simulink model "sampleModel1000"  (R2022a)
settings: Solver=VariableStepAuto  StartTime=0.0  StopTime=10.0  RelTol=1e-3
undefined symbols (not defined in the file): DiscIntNeverNeededParam, magnitude, Newton, Raphson
libraries: simulink x216, slpidlib x76
(part 3 of 10)

== system sampleModel1000/cfblk162 ==
  cfblk1 : Inport
  cfblk14 : Inport  Port=2
  cfblk10 : Subsystem
  cfblk11 : Subsystem
  cfblk12 : Subsystem
  cfblk13 : Subsystem
  cfblk{16..19} (4 alike) : Delay  SampleTime=1
  cfblk3 : slpidlib/PID Controller (2DOF)  Controller=PID  Form=Parallel  TimeDomain=Discrete-time  UseExternalTs=off  SampleTime=1  IntegratorMethod=Forward Euler  FilterMethod=Forward Euler  ControllerParametersSource=internal  P=1  I=1  UseKiTs=off  D=0  N=100  UseFilter=on  b=1  c=1  TunerSelectOption=Transfer Function Based (PID Tuner App)  InitialConditionSource=internal  InitialConditionForIntegrator=0  InitialConditionForFilter=0  DifferentiatorICPrevScaledInput=0  ExternalReset=none  TrackingMode=off  Kt=1  LimitOutput=off  SatLimitsSource=internal  UpperSaturationLimit=inf  LowerSaturationLimit=-inf  LinearizeAsGain=off  AntiWindupMode=none  Kb=1  POutMin=[]  POutMax=[]  IOutMin=[]  IOutMax=[]  DOutMin=[]  DOutMax=[]  NOutMin=[]  NOutMax=[]  bOutMin=[]  bOutMax=[]  cOutMin=[]  cOutMax=[]  SumOutMin=[]  SumOutMax=[]  SaturationOutMin=[]  SaturationOutMax=[]  PParamMin=[]  PParamMax=[]  IParamMin=[]  IParamMax=[]  DParamMin=[]  DParamMax=[]  NParamMin=[]  NParamMax=[]  bParamMin=[]  bParamMax=[]  cParamMin=[]  cParamMax=[]  KbParamMin=[]  KbParamMax=[]  KtParamMin=[]  KtParamMax=[]  KbOutMin=[]  KbOutMax=[]  KtOutMin=[]  KtOutMax=[]  IntegratorOutMin=[]  IntegratorOutMax=[]  FilterOutMin=[]  FilterOutMax=[]  SumI1OutMin=[]  SumI1OutMax=[]  SumI2OutMin=[]  SumI2OutMax=[]  SumI3OutMin=[]  SumI3OutMax=[]  SumI4OutMin=[]  SumI4OutMax=[]  SumDOutMin=[]  SumDOutMax=[]  Sum1OutMin=[]  Sum1OutMax=[]  Sum2OutMin=[]  Sum2OutMax=[]  Sum3OutMin=[]  Sum3OutMax=[]  DifferentiatorOutMin=[]  DifferentiatorOutMax=[]  FilterDiffOutCoefMin=[]  FilterDiffOutCoefMax=[]  ReciprocalOutMin=[]  ReciprocalOutMax=[]  SumDenOutMin=[]  SumDenOutMax=[]  SumNumOutMin=[]  SumNumOutMax=[]  DivideOutMin=[]  DivideOutMax=[]  UdiffTsProdOutMin=[]  UdiffTsProdOutMax=[]  NTsProdOutMin=[]  NTsProdOutMax=[]  UintegralTsProdOutMin=[]  UintegralTsProdOutMax=[]  UngainTsProdOutMin=[]  UngainTsProdOutMax=[]  IntegratorContinuousStateAttributes=''  IntegratorStateMustResolveToSignalObject=off  IntegratorRTWStateStorageClass=Auto  FilterContinuousStateAttributes=''  FilterStateMustResolveToSignalObject=off  FilterRTWStateStorageClass=Auto  ParallelPVariant=InternalParameters  IdealPVariant=Disabled  IVariant=InternalParameters  DVariant=InternalParameters  bVariant=InternalParameters  cVariant=InternalParameters  IntegratorVariant=Discrete  SatVariant=Disabled  AWVariant=Passthrough  PCopyVariant=Disabled  TRVariant=Disabled  FdbkBlocksVariant=Forward  IdealPFdbkVariant=Disabled  SatFdbkVariant=Disabled  DerivativeFilterVariant=ForwardEulerFilter  NVariant=InternalParameters  NCopyVariant=Disabled  FilterICVariant=InternalICsFilter  IntegratorICVariant=InternalICs  ExternalResetVariant=Disabled  TRSumVariant=Passthrough  SumFdbkVariant=Disabled  SumVariant=Sum_PID  TsampFilterVariant=InternalTs  TsampNgainVariant=Passthrough  TsampIntegralVariant=Passthrough  ExternalSaturationOutDataTypeStr=Inherit: Same as second input
      settings: SourceProductBaseCode=SL
  cfblk4 : simulink/Discrete/Transfer Fcn First Order  PoleZ=0.95  ICPrevOutput=0.0  DoSatur=off
  cfblk5 : ComplexToMagnitudeAngle
  cfblk6 : Sum  Inputs=+-
  cfblk7 : Abs  SaturateOnIntegerOverflow=off
  cfblk8 : Rounding
  cfblk9 : Constant  Value=[225906652.287028]  SampleTime=1
  cfblk2 : Outport
  cfblk15 : Outport  Port=2
  wires:
  cfblk13/1(cfblk2) -> cfblk3/1, cfblk11/4(cfblk13)
  cfblk10/1(cfblk2) -> cfblk8/1
  cfblk6/1 -> cfblk15/1
  cfblk3/1 -> cfblk4/1
  cfblk7/1 -> cfblk5/1, cfblk18/1
  cfblk9/1 -> cfblk3/2
  cfblk1/1 -> cfblk6/1, cfblk12/3(cfblk8)
  cfblk12/1(cfblk2) -> cfblk13/2(cfblk7)
  cfblk10/2(cfblk15) -> cfblk11/1(cfblk1)
  cfblk8/1 -> cfblk2/1
  cfblk5/2 -> cfblk11/2(cfblk11), cfblk11/3(cfblk12)
  cfblk4/1 -> cfblk10/2(cfblk13)
  cfblk14/1 -> cfblk13/3(cfblk8), cfblk12/4(cfblk9)
  cfblk10/3(cfblk16) -> cfblk7/1
  cfblk12/2(cfblk10) -> cfblk10/3(cfblk14)
  cfblk12/3(cfblk11) -> cfblk6/2
  cfblk11/1(cfblk2) -> cfblk16/1
  cfblk16/1 -> cfblk12/2(cfblk7)
  cfblk11/2(cfblk14) -> cfblk17/1
  cfblk17/1 -> cfblk10/1(cfblk1)
  cfblk18/1 -> cfblk12/1(cfblk1)
  cfblk5/1 -> cfblk19/1
  cfblk19/1 -> cfblk13/1(cfblk1)

== system sampleModel1000/cfblk163 ==
  cfblk1 : Inport
  cfblk10 : Delay  SampleTime=1
  cfblk11 : Delay  SampleTime=1
  cfblk3 : slpidlib/PID Controller (2DOF)  Controller=PID  Form=Parallel  TimeDomain=Discrete-time  UseExternalTs=off  SampleTime=1  IntegratorMethod=Forward Euler  FilterMethod=Forward Euler  ControllerParametersSource=internal  P=1  I=1  UseKiTs=off  D=0  N=100  UseFilter=on  b=1  c=1  TunerSelectOption=Transfer Function Based (PID Tuner App)  InitialConditionSource=internal  InitialConditionForIntegrator=0  InitialConditionForFilter=0  DifferentiatorICPrevScaledInput=0  ExternalReset=none  TrackingMode=off  Kt=1  LimitOutput=off  SatLimitsSource=internal  UpperSaturationLimit=inf  LowerSaturationLimit=-inf  LinearizeAsGain=off  AntiWindupMode=none  Kb=1  POutMin=[]  POutMax=[]  IOutMin=[]  IOutMax=[]  DOutMin=[]  DOutMax=[]  NOutMin=[]  NOutMax=[]  bOutMin=[]  bOutMax=[]  cOutMin=[]  cOutMax=[]  SumOutMin=[]  SumOutMax=[]  SaturationOutMin=[]  SaturationOutMax=[]  PParamMin=[]  PParamMax=[]  IParamMin=[]  IParamMax=[]  DParamMin=[]  DParamMax=[]  NParamMin=[]  NParamMax=[]  bParamMin=[]  bParamMax=[]  cParamMin=[]  cParamMax=[]  KbParamMin=[]  KbParamMax=[]  KtParamMin=[]  KtParamMax=[]  KbOutMin=[]  KbOutMax=[]  KtOutMin=[]  KtOutMax=[]  IntegratorOutMin=[]  IntegratorOutMax=[]  FilterOutMin=[]  FilterOutMax=[]  SumI1OutMin=[]  SumI1OutMax=[]  SumI2OutMin=[]  SumI2OutMax=[]  SumI3OutMin=[]  SumI3OutMax=[]  SumI4OutMin=[]  SumI4OutMax=[]  SumDOutMin=[]  SumDOutMax=[]  Sum1OutMin=[]  Sum1OutMax=[]  Sum2OutMin=[]  Sum2OutMax=[]  Sum3OutMin=[]  Sum3OutMax=[]  DifferentiatorOutMin=[]  DifferentiatorOutMax=[]  FilterDiffOutCoefMin=[]  FilterDiffOutCoefMax=[]  ReciprocalOutMin=[]  ReciprocalOutMax=[]  SumDenOutMin=[]  SumDenOutMax=[]  SumNumOutMin=[]  SumNumOutMax=[]  DivideOutMin=[]  DivideOutMax=[]  UdiffTsProdOutMin=[]  UdiffTsProdOutMax=[]  NTsProdOutMin=[]  NTsProdOutMax=[]  UintegralTsProdOutMin=[]  UintegralTsProdOutMax=[]  UngainTsProdOutMin=[]  UngainTsProdOutMax=[]  IntegratorContinuousStateAttributes=''  IntegratorStateMustResolveToSignalObject=off  IntegratorRTWStateStorageClass=Auto  FilterContinuousStateAttributes=''  FilterStateMustResolveToSignalObject=off  FilterRTWStateStorageClass=Auto  ParallelPVariant=InternalParameters  IdealPVariant=Disabled  IVariant=InternalParameters  DVariant=InternalParameters  bVariant=InternalParameters  cVariant=InternalParameters  IntegratorVariant=Discrete  SatVariant=Disabled  AWVariant=Passthrough  PCopyVariant=Disabled  TRVariant=Disabled  FdbkBlocksVariant=Forward  IdealPFdbkVariant=Disabled  SatFdbkVariant=Disabled  DerivativeFilterVariant=ForwardEulerFilter  NVariant=InternalParameters  NCopyVariant=Disabled  FilterICVariant=InternalICsFilter  IntegratorICVariant=InternalICs  ExternalResetVariant=Disabled  TRSumVariant=Passthrough  SumFdbkVariant=Disabled  SumVariant=Sum_PID  TsampFilterVariant=InternalTs  TsampNgainVariant=Passthrough  TsampIntegralVariant=Passthrough  ExternalSaturationOutDataTypeStr=Inherit: Same as second input
      settings: SourceProductBaseCode=SL
  cfblk4 : DiscreteFir  SampleTime=1
  cfblk5 : ComplexToRealImag
  cfblk6 : DotProduct  OutDataTypeStr=Inherit: Inherit via internal rule
  cfblk7 : Subsystem
  cfblk8 : Subsystem
  cfblk9 : Delay  SampleTime=1
  cfblk2 : Outport
  wires:
  cfblk3/1 -> cfblk8/1(cfblk1)
  cfblk6/1 -> cfblk7/1(cfblk1), cfblk3/2
  cfblk1/1 -> cfblk6/1
  cfblk4/1 -> cfblk2/1
  cfblk7/1(cfblk2) -> cfblk8/2(cfblk6)
  cfblk8/1(cfblk2) -> cfblk5/1
  cfblk7/2(cfblk8) -> cfblk4/1
  cfblk7/3(cfblk9) -> cfblk3/1
  cfblk5/1 -> cfblk9/1
  cfblk9/1 -> cfblk6/2
  cfblk5/2 -> cfblk10/1
  cfblk10/1 -> cfblk8/3(cfblk7)
  cfblk8/2(cfblk8) -> cfblk11/1
  cfblk11/1 -> cfblk7/2(cfblk7)

== system sampleModel1000/cfblk164 ==
  cfblk1 : Inport
  cfblk8 : Inport  Port=2
  cfblk10 : Subsystem  TreatAsAtomicUnit=on
  cfblk11 : Subsystem  TreatAsAtomicUnit=on
  cfblk12 : Delay  SampleTime=1
  cfblk3 : simulink/Math Operations/MinMax Running Resettable  Function=min  vinit=0.0
  cfblk4 : Sqrt  Operator=rSqrt  AlgorithmType=Newton-Raphson
  cfblk5 : Constant  Value=[165198451.789019]  SampleTime=1
  cfblk6 : Subsystem
  cfblk7 : If  IfExpression=u1 >= 0  SampleTime=1
  cfblk2 : Outport
  cfblk9 : Outport  Port=2
  wires:
  cfblk3/1 -> cfblk2/1
  cfblk8/1 -> cfblk4/1
  cfblk5/1 -> cfblk9/1, cfblk10/2(cfblk9)
  cfblk6/1(cfblk2) -> cfblk11/1(cfblk1)
  cfblk6/2(cfblk10) -> cfblk7/1
  cfblk6/3(cfblk11) -> cfblk3/1
  cfblk1/1 -> cfblk3/2
  cfblk4/1 -> cfblk6/2(cfblk9), cfblk10/3(cfblk10)
  cfblk11/1(cfblk2) -> cfblk10/1(cfblk1)
  cfblk7/1 -> cfblk10/Action
  cfblk7/2 -> cfblk11/Action
  cfblk10/1(cfblk2) -> cfblk12/1
  cfblk12/1 -> cfblk6/1(cfblk1)

== system sampleModel1000/cfblk165 ==
  cfblk1 : Inport
  cfblk10 : Subsystem
  cfblk11 : Subsystem
  cfblk12 : Subsystem
  cfblk13 : Subsystem
  cfblk15 : Delay  SampleTime=1
  cfblk3 : DiscreteStateSpace
  cfblk4 : Delay  SampleTime=1
  cfblk5 : Sum  Inputs=+
  cfblk6 : Constant  Value=[-942559068.084859]  SampleTime=1
  cfblk7 : Constant  Value=[883886855.435224]  SampleTime=1
  cfblk8 : Constant  Value=[497965959.676924]  SampleTime=1
  cfblk9 : Constant  Value=[-864930801.055590]  SampleTime=1
  cfblk2 : Outport
  cfblk14 : Outport  Port=2
  wires:
  cfblk7/1 -> cfblk5/1
  cfblk4/1 -> cfblk12/1(cfblk1)
  cfblk1/1 -> cfblk10/1(cfblk1)
  cfblk5/1 -> cfblk10/2(cfblk6)
  cfblk3/1 -> cfblk13/1(cfblk1), cfblk13/2(cfblk9)
  cfblk9/1 -> cfblk10/3(cfblk7)
  cfblk11/1(cfblk2) -> cfblk3/1
  cfblk6/1 -> cfblk11/1(cfblk1), cfblk2/1
  cfblk12/1(cfblk2) -> cfblk14/1
  cfblk8/1 -> cfblk11/2(cfblk16)
  cfblk12/2(cfblk16) -> cfblk11/3(cfblk17)
  cfblk10/1(cfblk2) -> cfblk4/1
  cfblk13/1(cfblk2) -> cfblk15/1
  cfblk15/1 -> cfblk12/2(cfblk15)

== system sampleModel1000/cfblk166 ==
  cfblk1 : Inport
  cfblk10 : Subsystem
  cfblk11 : Subsystem
  cfblk{12..16} (5 alike) : Delay  SampleTime=1
  cfblk3 : simulink/Discrete/Transfer Fcn Real Zero  ZeroZ=0.75  ICPrevInput=0.0  DoSatur=off
      settings: SourceProductBaseCode=SL
  cfblk4 : simulink/Discrete/Transfer Fcn First Order  PoleZ=0.95  ICPrevOutput=0.0  DoSatur=off
  cfblk5 : slpidlib/PID Controller (2DOF)  Controller=PID  Form=Parallel  TimeDomain=Discrete-time  UseExternalTs=off  SampleTime=1  IntegratorMethod=Forward Euler  FilterMethod=Forward Euler  ControllerParametersSource=internal  P=1  I=1  UseKiTs=off  D=0  N=100  UseFilter=on  b=1  c=1  TunerSelectOption=Transfer Function Based (PID Tuner App)  InitialConditionSource=internal  InitialConditionForIntegrator=0  InitialConditionForFilter=0  DifferentiatorICPrevScaledInput=0  ExternalReset=none  TrackingMode=off  Kt=1  LimitOutput=off  SatLimitsSource=internal  UpperSaturationLimit=inf  LowerSaturationLimit=-inf  LinearizeAsGain=off  AntiWindupMode=none  Kb=1  POutMin=[]  POutMax=[]  IOutMin=[]  IOutMax=[]  DOutMin=[]  DOutMax=[]  NOutMin=[]  NOutMax=[]  bOutMin=[]  bOutMax=[]  cOutMin=[]  cOutMax=[]  SumOutMin=[]  SumOutMax=[]  SaturationOutMin=[]  SaturationOutMax=[]  PParamMin=[]  PParamMax=[]  IParamMin=[]  IParamMax=[]  DParamMin=[]  DParamMax=[]  NParamMin=[]  NParamMax=[]  bParamMin=[]  bParamMax=[]  cParamMin=[]  cParamMax=[]  KbParamMin=[]  KbParamMax=[]  KtParamMin=[]  KtParamMax=[]  KbOutMin=[]  KbOutMax=[]  KtOutMin=[]  KtOutMax=[]  IntegratorOutMin=[]  IntegratorOutMax=[]  FilterOutMin=[]  FilterOutMax=[]  SumI1OutMin=[]  SumI1OutMax=[]  SumI2OutMin=[]  SumI2OutMax=[]  SumI3OutMin=[]  SumI3OutMax=[]  SumI4OutMin=[]  SumI4OutMax=[]  SumDOutMin=[]  SumDOutMax=[]  Sum1OutMin=[]  Sum1OutMax=[]  Sum2OutMin=[]  Sum2OutMax=[]  Sum3OutMin=[]  Sum3OutMax=[]  DifferentiatorOutMin=[]  DifferentiatorOutMax=[]  FilterDiffOutCoefMin=[]  FilterDiffOutCoefMax=[]  ReciprocalOutMin=[]  ReciprocalOutMax=[]  SumDenOutMin=[]  SumDenOutMax=[]  SumNumOutMin=[]  SumNumOutMax=[]  DivideOutMin=[]  DivideOutMax=[]  UdiffTsProdOutMin=[]  UdiffTsProdOutMax=[]  NTsProdOutMin=[]  NTsProdOutMax=[]  UintegralTsProdOutMin=[]  UintegralTsProdOutMax=[]  UngainTsProdOutMin=[]  UngainTsProdOutMax=[]  IntegratorContinuousStateAttributes=''  IntegratorStateMustResolveToSignalObject=off  IntegratorRTWStateStorageClass=Auto  FilterContinuousStateAttributes=''  FilterStateMustResolveToSignalObject=off  FilterRTWStateStorageClass=Auto  ParallelPVariant=InternalParameters  IdealPVariant=Disabled  IVariant=InternalParameters  DVariant=InternalParameters  bVariant=InternalParameters  cVariant=InternalParameters  IntegratorVariant=Discrete  SatVariant=Disabled  AWVariant=Passthrough  PCopyVariant=Disabled  TRVariant=Disabled  FdbkBlocksVariant=Forward  IdealPFdbkVariant=Disabled  SatFdbkVariant=Disabled  DerivativeFilterVariant=ForwardEulerFilter  NVariant=InternalParameters  NCopyVariant=Disabled  FilterICVariant=InternalICsFilter  IntegratorICVariant=InternalICs  ExternalResetVariant=Disabled  TRSumVariant=Passthrough  SumFdbkVariant=Disabled  SumVariant=Sum_PID  TsampFilterVariant=InternalTs  TsampNgainVariant=Passthrough  TsampIntegralVariant=Passthrough  ExternalSaturationOutDataTypeStr=Inherit: Same as second input
      settings: SourceProductBaseCode=SL
  cfblk6 : Abs  SaturateOnIntegerOverflow=off
  cfblk7 : Reshape
  cfblk8 : Subsystem
  cfblk9 : Subsystem
  cfblk2 : Outport
  wires:
  cfblk1/1 -> cfblk2/1
  cfblk3/1 -> cfblk10/1(cfblk1)
  cfblk4/1 -> cfblk8/1(cfblk1), cfblk8/2(cfblk7)
  cfblk11/1(cfblk2) -> cfblk4/1
  cfblk10/1(cfblk2) -> cfblk7/1, cfblk11/3(cfblk13)
  cfblk5/1 -> cfblk6/1
  cfblk8/1(cfblk2) -> cfblk9/1(cfblk1), cfblk5/2
  cfblk7/1 -> cfblk12/1
  cfblk12/1 -> cfblk10/2(cfblk7)
  cfblk9/1(cfblk2) -> cfblk13/1
  cfblk13/1 -> cfblk11/1(cfblk1)
  cfblk9/2(cfblk13) -> cfblk14/1
  cfblk14/1 -> cfblk11/2(cfblk12)
  cfblk6/1 -> cfblk15/1
  cfblk15/1 -> cfblk5/1
  cfblk11/2(cfblk14) -> cfblk16/1
  cfblk16/1 -> cfblk3/1

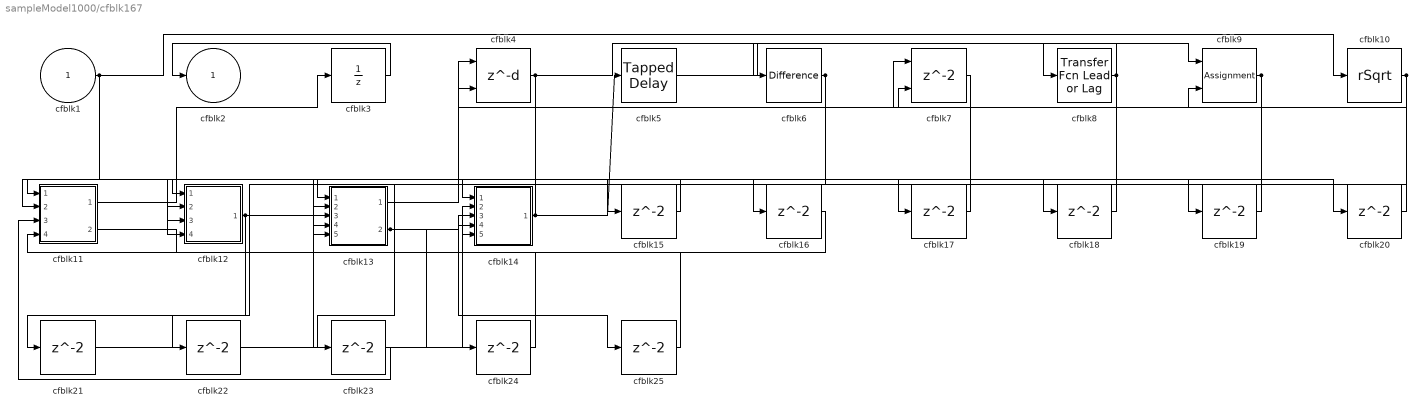
== system sampleModel1000/cfblk167 ==
  cfblk1 : Inport
  cfblk10 : Sqrt  Operator=rSqrt  AlgorithmType=Newton-Raphson
  cfblk11 : Subsystem
  cfblk12 : Subsystem
  cfblk13 : Subsystem
  cfblk14 : Subsystem
  cfblk{15..25} (11 alike) : Delay  SampleTime=1
  cfblk3 : UnitDelay  HasFrameUpgradeWarning=on
  cfblk4 : Delay  DelayLengthSource=Input port  SampleTime=1
      settings: InputPortMap=u0,p1
  cfblk5 : simulink/Discrete/Tapped Delay  vinit=0.0  samptime=-1  NumDelays=1  DelayOrder=Oldest  includeCurrent=off
  cfblk6 : simulink/Discrete/Difference  ICPrevInput=0.0  OutMin=[]  OutMax=[]  OutDataTypeStr=Inherit: Inherit via back propagation  OutDataType=fixdt(1, 16)  OutScaling=2^-10  DoSatur=off
  cfblk7 : Delay  ShowEnablePort=on  SampleTime=1
      settings: InputPortMap=u0,e6
  cfblk8 : simulink/Discrete/Transfer Fcn Lead or Lag  PoleZ=0.95  ZeroZ=0.75  ICPrevOutput=0.0  ICPrevInput=0.0  DoSatur=off
      settings: SourceProductBaseCode=SL
  cfblk9 : Assignment  DiagnosticForDimensions=Warning  IndexOptions=Index vector (dialog)  Indices=1  OutputSizes=1
  cfblk2 : Outport
  wires:
  cfblk6/1 -> cfblk13/4(cfblk12), cfblk13/5(cfblk13), cfblk15/1, cfblk16/1
  cfblk4/1 -> cfblk9/1, cfblk22/1, cfblk23/1
  cfblk14/1(cfblk2) -> cfblk5/1, cfblk12/1(cfblk1)
  cfblk12/1(cfblk2) -> cfblk18/1, cfblk19/1, cfblk20/1, cfblk21/1
  cfblk5/1 -> cfblk8/1
  cfblk3/1 -> cfblk2/1
  cfblk13/1(cfblk2) -> cfblk4/2
  cfblk8/1 -> cfblk6/1, cfblk12/2(cfblk7), cfblk12/3(cfblk8)
  cfblk1/1 -> cfblk10/1, cfblk11/2(cfblk13)
  cfblk11/1(cfblk2) -> cfblk3/1
  cfblk9/1 -> cfblk12/4(cfblk9), cfblk17/1
  cfblk11/2(cfblk16) -> cfblk14/2(cfblk9)
  cfblk13/2(cfblk14) -> cfblk24/1, cfblk25/1
  cfblk7/1 -> cfblk11/1(cfblk1)
  cfblk10/1 -> cfblk7/2, cfblk13/3(cfblk11)
  cfblk15/1 -> cfblk14/1(cfblk1)
  cfblk16/1 -> cfblk14/4(cfblk11)
  cfblk17/1 -> cfblk7/1
  cfblk18/1 -> cfblk4/1
  cfblk19/1 -> cfblk13/1(cfblk1)
  cfblk20/1 -> cfblk9/2
  cfblk21/1 -> cfblk14/5(cfblk12)
  cfblk22/1 -> cfblk13/2(cfblk10)
  cfblk23/1 -> cfblk11/3(cfblk14)
  cfblk24/1 -> cfblk14/3(cfblk10)
  cfblk25/1 -> cfblk11/4(cfblk15)

== system sampleModel1000/cfblk172 ==
  cfblk1 : Inport
  cfblk8 : Inport  Port=2
  cfblk9 : Inport  Port=3
  Action Port : ActionPort  ActionPortLabel=if(u1 >= 0)
  cfblk13 : Delay
  cfblk14 : Delay
  cfblk3 : Delay  DelayLengthSource=Input port
      settings: InputPortMap=u0,p1
  cfblk4 : DotProduct  OutDataTypeStr=Inherit: Inherit via internal rule
  cfblk5 : Bias  Bias=[-981896496.671073]  SaturateOnIntegerOverflow=off
  cfblk6 : Subsystem
  cfblk7 : Subsystem
  cfblk2 : Outport
  cfblk10 : Outport  Port=2
  cfblk11 : Outport  Port=3
  cfblk12 : Outport  Port=4
  wires:
  cfblk3/1 -> cfblk12/1, cfblk6/1(cfblk1)
  cfblk9/1 -> cfblk5/1
  cfblk5/1 -> cfblk4/1, cfblk6/4(cfblk11)
  cfblk6/2(cfblk12) -> cfblk4/2
  cfblk7/1(cfblk2) -> cfblk10/1
  cfblk6/3(cfblk13) -> cfblk11/1, cfblk7/3(cfblk15), cfblk7/4(cfblk16)
  cfblk8/1 -> cfblk3/2, cfblk7/2(cfblk14), cfblk6/2(cfblk9)
  cfblk1/1 -> cfblk2/1
  cfblk4/1 -> cfblk7/1(cfblk1), cfblk14/1
  cfblk6/1(cfblk2) -> cfblk13/1
  cfblk13/1 -> cfblk3/1
  cfblk14/1 -> cfblk6/3(cfblk10)

== system sampleModel1000/cfblk173 ==
  cfblk1 : Inport
  cfblk7 : Inport  Port=2
  cfblk8 : Inport  Port=3
  Action Port : ActionPort  ActionPortLabel=else
  cfblk3 : simulink/Discrete/Transfer Fcn Lead or Lag  PoleZ=0.95  ZeroZ=0.75  ICPrevOutput=0.0  ICPrevInput=0.0  DoSatur=off
      settings: SourceProductBaseCode=SL
  cfblk4 : PermuteDimensions
  cfblk5 : Assignment  DiagnosticForDimensions=Warning  IndexOptions=Index vector (dialog)  Indices=1  OutputSizes=1
  cfblk6 : Math
  cfblk9 : Delay
  cfblk2 : Outport
  wires:
  cfblk1/1 -> cfblk6/1
  cfblk7/1 -> cfblk2/1
  cfblk4/1 -> cfblk5/1
  cfblk6/1 -> cfblk3/1
  cfblk8/1 -> cfblk5/2
  cfblk5/1 -> cfblk9/1
  cfblk9/1 -> cfblk4/1

== system sampleModel1000/cfblk174 ==
  cfblk1 : Inport
  Action Port : ActionPort  ActionPortLabel=if(u1 >= 0)
  cfblk10 : Delay
  cfblk11 : Delay
  cfblk3 : Rounding
  cfblk4 : Reshape
  cfblk5 : Polyval  Coefs=[ +2.081618890e-019, -1.441693666e-014, +4.719686976e-010, -8.536869453e-006, +1.621573104e-001, -8.087801117e+001 ]
  cfblk6 : simulink/Math Operations/Slider Gain  gain=1  low=0  high=2
  cfblk7 : Subsystem
  cfblk8 : Subsystem
  cfblk9 : Delay
  cfblk2 : Outport
  wires:
  cfblk5/1 -> cfblk4/1
  cfblk3/1 -> cfblk5/1
  cfblk7/1(cfblk2) -> cfblk8/1(cfblk1)
  cfblk4/1 -> cfblk6/1
  cfblk6/1 -> cfblk7/3(cfblk8)
  cfblk1/1 -> cfblk2/1
  cfblk8/1(cfblk2) -> cfblk9/1
  cfblk9/1 -> cfblk7/1(cfblk1)
  cfblk8/2(cfblk12) -> cfblk10/1
  cfblk10/1 -> cfblk3/1
  cfblk8/3(cfblk13) -> cfblk11/1
  cfblk11/1 -> cfblk7/2(cfblk7)

== system sampleModel1000/cfblk175 ==
  cfblk1 : Inport
  cfblk7 : Inport  Port=2
  Action Port : ActionPort  ActionPortLabel=else
  cfblk10 : Subsystem  TreatAsAtomicUnit=on
  cfblk{11..16} (6 alike) : Delay
  cfblk3 : Product  Inputs=*
  cfblk4 : Subsystem
  cfblk5 : Subsystem
  cfblk6 : If  IfExpression=u1 >= 0  SampleTime=1
  cfblk9 : Subsystem  TreatAsAtomicUnit=on
  cfblk2 : Outport
  cfblk8 : Outport  Port=2
  wires:
  cfblk10/1(cfblk2) -> cfblk3/1
  cfblk1/1 -> cfblk8/1, cfblk4/4(cfblk10)
  cfblk7/1 -> cfblk9/1(cfblk1), cfblk5/2(cfblk13)
  cfblk9/1(cfblk2) -> cfblk11/1, cfblk12/1
  cfblk4/1(cfblk2) -> cfblk9/2(cfblk13)
  cfblk3/1 -> cfblk2/1, cfblk5/3(cfblk14), cfblk13/1, cfblk14/1
  cfblk10/2(cfblk7) -> cfblk5/1(cfblk1), cfblk9/4(cfblk15)
  cfblk4/2(cfblk11) -> cfblk6/1, cfblk5/4(cfblk15)
  cfblk6/1 -> cfblk9/Action
  cfblk6/2 -> cfblk10/Action
  cfblk11/1 -> cfblk4/1(cfblk1)
  cfblk12/1 -> cfblk4/2(cfblk8)
  cfblk13/1 -> cfblk9/3(cfblk14)
  cfblk14/1 -> cfblk4/3(cfblk9)
  cfblk5/1(cfblk2) -> cfblk15/1
  cfblk15/1 -> cfblk10/1(cfblk1)
  cfblk5/2(cfblk16) -> cfblk16/1
  cfblk16/1 -> cfblk10/2(cfblk6)

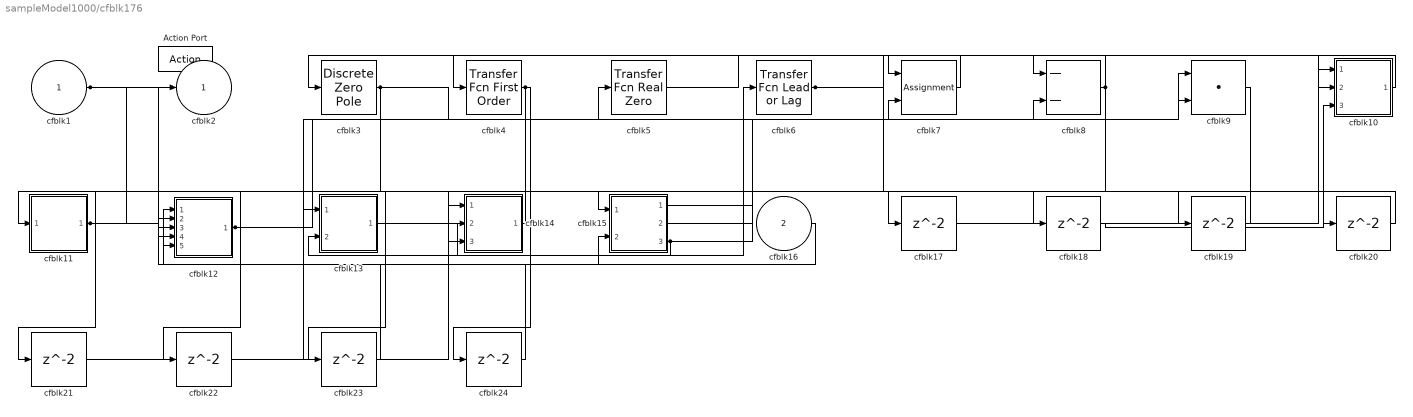
== system sampleModel1000/cfblk176 ==
  cfblk1 : Inport
  cfblk16 : Inport  Port=2
  Action Port : ActionPort  ActionPortLabel=if(u1 >= 0)
  cfblk10 : Subsystem
  cfblk11 : Subsystem
  cfblk12 : Subsystem
  cfblk13 : Subsystem
  cfblk14 : Subsystem
  cfblk15 : Subsystem
  cfblk{17..24} (8 alike) : Delay
  cfblk3 : DiscreteZeroPole  Poles=[0 0.5]  Gain=1  SampleTime=-1
  cfblk4 : simulink/Discrete/Transfer Fcn First Order  PoleZ=0.95  ICPrevOutput=0.0  DoSatur=off
  cfblk5 : simulink/Discrete/Transfer Fcn Real Zero  ZeroZ=0.75  ICPrevInput=0.0  DoSatur=off
      settings: SourceProductBaseCode=SL
  cfblk6 : simulink/Discrete/Transfer Fcn Lead or Lag  PoleZ=0.95  ZeroZ=0.75  ICPrevOutput=0.0  ICPrevInput=0.0  DoSatur=off
      settings: SourceProductBaseCode=SL
  cfblk7 : Assignment  DiagnosticForDimensions=Warning  IndexOptions=Index vector (dialog)  Indices=1  OutputSizes=1
  cfblk8 : Sum  Inputs=--
  cfblk9 : DotProduct  OutDataTypeStr=Inherit: Inherit via internal rule
  cfblk2 : Outport
  wires:
  cfblk11/1(cfblk2) -> cfblk2/1, cfblk15/2(cfblk8)
  cfblk3/1 -> cfblk9/2, cfblk22/1
  cfblk13/1(cfblk2) -> cfblk6/1
  cfblk7/1 -> cfblk3/1
  cfblk14/1(cfblk2) -> cfblk11/1(cfblk1)
  cfblk16/1 -> cfblk12/1(cfblk1)
  cfblk12/1(cfblk2) -> cfblk5/1, cfblk7/2, cfblk8/2
  cfblk6/1 -> cfblk8/1, cfblk20/1
  cfblk4/1 -> cfblk14/2(cfblk12), cfblk24/1
  cfblk5/1 -> cfblk10/2(cfblk11)
  cfblk1/1 -> cfblk12/2(cfblk10), cfblk14/3(cfblk13)
  cfblk10/1(cfblk2) -> cfblk4/1
  cfblk15/3(cfblk10) -> cfblk9/1, cfblk13/2(cfblk15)
  cfblk8/1 -> cfblk7/1, cfblk21/1, cfblk23/1
  cfblk15/1(cfblk2) -> cfblk17/1
  cfblk17/1 -> cfblk10/1(cfblk1)
  cfblk15/2(cfblk9) -> cfblk18/1
  cfblk18/1 -> cfblk10/3(cfblk12)
  cfblk9/1 -> cfblk19/1
  cfblk19/1 -> cfblk12/3(cfblk11)
  cfblk20/1 -> cfblk15/1(cfblk1)
  cfblk21/1 -> cfblk13/1(cfblk1)
  cfblk22/1 -> cfblk14/1(cfblk1)
  cfblk23/1 -> cfblk12/4(cfblk12)
  cfblk24/1 -> cfblk12/5(cfblk13)

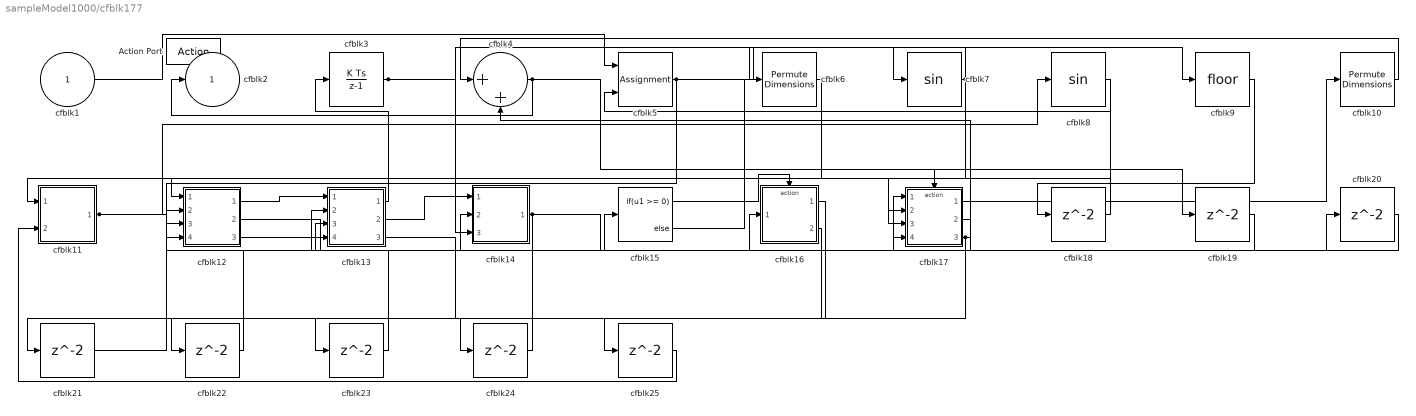
== system sampleModel1000/cfblk177 ==
  cfblk1 : Inport
  Action Port : ActionPort  ActionPortLabel=else
  cfblk10 : PermuteDimensions
  cfblk11 : Subsystem
  cfblk12 : Subsystem
  cfblk13 : Subsystem
  cfblk14 : Subsystem
  cfblk15 : If  IfExpression=u1 >= 0  SampleTime=1
  cfblk16 : Subsystem  TreatAsAtomicUnit=on
  cfblk17 : Subsystem  TreatAsAtomicUnit=on
  cfblk{18..25} (8 alike) : Delay
  cfblk3 : DiscreteIntegrator  SampleTime=-1  ICPrevOutput=DiscIntNeverNeededParam  ICPrevScaledInput=DiscIntNeverNeededParam
  cfblk4 : Sum  Inputs=|++
  cfblk5 : Assignment  DiagnosticForDimensions=Warning  IndexOptions=Index vector (dialog)  Indices=1  OutputSizes=1
  cfblk6 : PermuteDimensions
  cfblk7 : Trigonometry
  cfblk8 : Trigonometry
  cfblk9 : Rounding
  cfblk2 : Outport
  wires:
  cfblk4/1 -> cfblk2/1, cfblk19/1
  cfblk5/1 -> cfblk7/1, cfblk17/3(cfblk10), cfblk12/4(cfblk14)
  cfblk8/1 -> cfblk12/1(cfblk1)
  cfblk10/1 -> cfblk4/1
  cfblk11/1(cfblk2) -> cfblk8/1, cfblk13/3(cfblk9)
  cfblk17/1(cfblk2) -> cfblk10/1
  cfblk13/1(cfblk2) -> cfblk3/1
  cfblk1/1 -> cfblk5/1
  cfblk13/2(cfblk11) -> cfblk14/1(cfblk1)
  cfblk3/1 -> cfblk9/1, cfblk17/2(cfblk9)
  cfblk14/1(cfblk2) -> cfblk20/1, cfblk23/1
  cfblk6/1 -> cfblk11/1(cfblk1)
  cfblk7/1 -> cfblk6/1, cfblk14/3(cfblk14)
  cfblk17/2(cfblk12) -> cfblk14/2(cfblk13)
  cfblk17/3(cfblk13) -> cfblk4/2, cfblk24/1
  cfblk12/1(cfblk2) -> cfblk13/1(cfblk1)
  cfblk12/2(cfblk15) -> cfblk15/1
  cfblk12/3(cfblk16) -> cfblk17/1(cfblk1)
  cfblk15/1 -> cfblk16/Action
  cfblk15/2 -> cfblk17/Action
  cfblk9/1 -> cfblk18/1
  cfblk18/1 -> cfblk5/2
  cfblk19/1 -> cfblk17/4(cfblk11)
  cfblk20/1 -> cfblk16/1(cfblk1)
  cfblk16/1(cfblk2) -> cfblk21/1
  cfblk21/1 -> cfblk12/2(cfblk12)
  cfblk16/2(cfblk16) -> cfblk22/1
  cfblk22/1 -> cfblk12/3(cfblk13)
  cfblk23/1 -> cfblk13/4(cfblk10)
  cfblk24/1 -> cfblk13/2(cfblk8)
  cfblk13/3(cfblk12) -> cfblk25/1
  cfblk25/1 -> cfblk11/2(cfblk7)

== system sampleModel1000/cfblk178 ==
  cfblk1 : Inport
  cfblk9 : Inport  Port=2
  Action Port : ActionPort  ActionPortLabel=if(u1 >= 0)
  cfblk{11..15} (5 alike) : Delay
  cfblk3 : DiscreteFir
  cfblk4 : UnitDelay  SampleTime=-1  HasFrameUpgradeWarning=on
  cfblk5 : Squeeze
  cfblk6 : Subsystem
  cfblk7 : Subsystem
  cfblk8 : Subsystem
  cfblk2 : Outport
  cfblk10 : Outport  Port=2
  wires:
  cfblk9/1 -> cfblk5/1
  cfblk5/1 -> cfblk10/1
  cfblk8/1(cfblk2) -> cfblk4/1
  cfblk7/1(cfblk2) -> cfblk11/1, cfblk12/1
  cfblk4/1 -> cfblk3/1, cfblk15/1
  cfblk3/1 -> cfblk2/1, cfblk6/2(cfblk7)
  cfblk1/1 -> cfblk8/1(cfblk1), cfblk8/4(cfblk15)
  cfblk6/1(cfblk2) -> cfblk7/1(cfblk1)
  cfblk6/3(cfblk9) -> cfblk7/2(cfblk12)
  cfblk11/1 -> cfblk6/1(cfblk1)
  cfblk12/1 -> cfblk8/5(cfblk16)
  cfblk6/2(cfblk8) -> cfblk13/1
  cfblk13/1 -> cfblk8/2(cfblk13)
  cfblk6/4(cfblk10) -> cfblk14/1
  cfblk14/1 -> cfblk8/3(cfblk14)
  cfblk15/1 -> cfblk8/6(cfblk17)

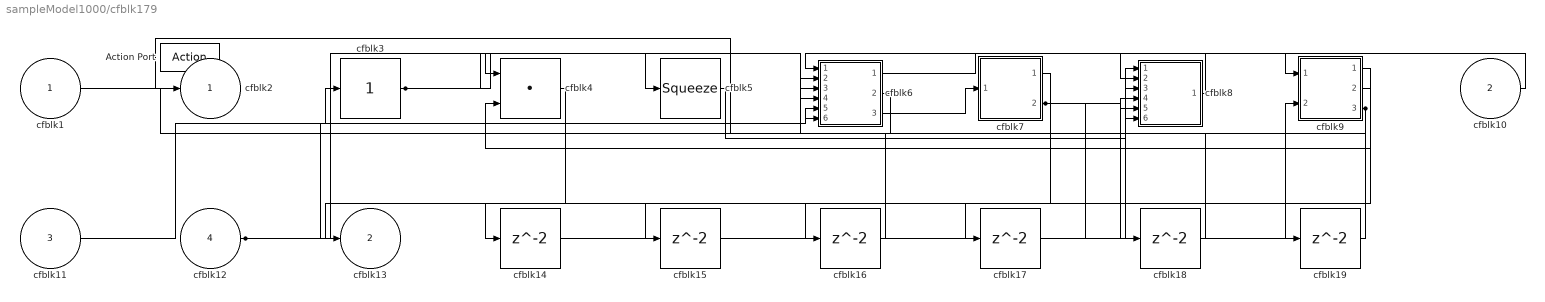
== system sampleModel1000/cfblk179 ==
  cfblk1 : Inport
  cfblk10 : Inport  Port=2
  cfblk11 : Inport  Port=3
  cfblk12 : Inport  Port=4
  Action Port : ActionPort  ActionPortLabel=else
  cfblk{14..19} (6 alike) : Delay
  cfblk3 : simulink/Math Operations/Slider Gain  gain=1  low=0  high=2
  cfblk4 : DotProduct  OutDataTypeStr=Inherit: Inherit via internal rule
  cfblk5 : Squeeze
  cfblk6 : Subsystem
  cfblk7 : Subsystem
  cfblk8 : Subsystem
  cfblk9 : Subsystem
  cfblk2 : Outport
  cfblk13 : Outport  Port=2
  wires:
  cfblk3/1 -> cfblk5/1, cfblk6/3(cfblk8)
  cfblk12/1 -> cfblk4/1, cfblk6/5(cfblk10), cfblk6/6(cfblk11)
  cfblk6/1(cfblk2) -> cfblk9/1(cfblk1)
  cfblk6/2(cfblk12) -> cfblk2/1
  cfblk5/1 -> cfblk8/1(cfblk1)
  cfblk9/1(cfblk2) -> cfblk4/2
  cfblk9/2(cfblk14) -> cfblk13/1
  cfblk11/1 -> cfblk3/1
  cfblk6/3(cfblk13) -> cfblk7/1(cfblk1)
  cfblk10/1 -> cfblk8/2(cfblk12)
  cfblk1/1 -> cfblk8/3(cfblk13)
  cfblk7/2(cfblk8) -> cfblk18/1, cfblk19/1
  cfblk8/1(cfblk2) -> cfblk6/1(cfblk1)
  cfblk9/3(cfblk15) -> cfblk15/1, cfblk16/1
  cfblk4/1 -> cfblk14/1
  cfblk14/1 -> cfblk9/2(cfblk13)
  cfblk15/1 -> cfblk8/6(cfblk16)
  cfblk16/1 -> cfblk6/2(cfblk7)
  cfblk7/1(cfblk2) -> cfblk17/1
  cfblk17/1 -> cfblk8/4(cfblk14)
  cfblk18/1 -> cfblk8/5(cfblk15)
  cfblk19/1 -> cfblk6/4(cfblk9)

== system sampleModel1000/cfblk125/cfblk10 ==
  cfblk1 : Inport
  cfblk13 : Inport  Port=2
  cfblk14 : Inport  Port=3
  cfblk15 : Inport  Port=4
  cfblk10 : Constant  Value=[781560997.885926]  SampleTime=1
  cfblk11 : Constant  Value=[-786325686.899081]  SampleTime=1
  cfblk12 : Constant  Value=[828386562.541228]  SampleTime=1
  cfblk3 : simulink/Discrete/Transfer Fcn Real Zero  ZeroZ=0.75  ICPrevInput=0.0  DoSatur=off
      settings: SourceProductBaseCode=SL
  cfblk4 : simulink/Discrete/Transfer Fcn First Order  PoleZ=0.95  ICPrevOutput=0.0  DoSatur=off
  cfblk5 : Delay  SampleTime=1
  cfblk6 : simulink/Math Operations/MinMax Running Resettable  Function=min  vinit=0.0
  cfblk7 : Assignment  DiagnosticForDimensions=Warning  IndexOptions=Index vector (dialog)  Indices=1  OutputSizes=1
  cfblk8 : Product  Inputs=*
  cfblk9 : Abs  SaturateOnIntegerOverflow=off
  cfblk2 : Outport
  cfblk16 : Outport  Port=2
  cfblk17 : Outport  Port=3
  wires:
  cfblk5/1 -> cfblk2/1
  cfblk10/1 -> cfblk8/1
  cfblk3/1 -> cfblk4/1
  cfblk1/1 -> cfblk6/1
  cfblk4/1 -> cfblk9/1
  cfblk8/1 -> cfblk6/2
  cfblk9/1 -> cfblk5/1
  cfblk6/1 -> cfblk7/1
  cfblk15/1 -> cfblk16/1
  cfblk13/1 -> cfblk17/1
  cfblk12/1 -> cfblk3/1
  cfblk11/1 -> cfblk7/2

== system sampleModel1000/cfblk125/cfblk11 ==
  cfblk1 : Inport
  cfblk10 : Constant  Value=[387348995.231708]  SampleTime=1
  cfblk12 : Delay  SampleTime=1
  cfblk3 : DiscreteZeroPole  Poles=[0 0.5]  Gain=1
  cfblk4 : Sum  Inputs=+-
  cfblk5 : DotProduct  OutDataTypeStr=Inherit: Inherit via internal rule
  cfblk6 : PermuteDimensions
  cfblk7 : MinMax  Inputs=2
  cfblk8 : ComplexToRealImag
  cfblk9 : ComplexToMagnitudeAngle
  cfblk2 : Outport
  cfblk11 : Outport  Port=2
  wires:
  cfblk4/1 -> cfblk11/1
  cfblk7/1 -> cfblk8/1
  cfblk6/1 -> cfblk2/1
  cfblk10/1 -> cfblk5/1
  cfblk5/1 -> cfblk3/1
  cfblk8/1 -> cfblk9/1
  cfblk9/1 -> cfblk5/2
  cfblk9/2 -> cfblk4/1, cfblk12/1
  cfblk3/1 -> cfblk6/1
  cfblk8/2 -> cfblk4/2
  cfblk1/1 -> cfblk7/1
  cfblk12/1 -> cfblk7/2

== system sampleModel1000/cfblk125/cfblk7 ==
  cfblk1 : Inport
  cfblk3 : DiscreteTransferFcn  SampleTime=1
  cfblk4 : ComplexToMagnitudeAngle
  cfblk5 : Signum
  cfblk6 : MinMax  Inputs=3
  cfblk7 : Constant  Value=[386930589.509342]  SampleTime=1
  cfblk8 : Constant  Value=[-598257646.830201]  SampleTime=1
  cfblk9 : Delay  SampleTime=1
  cfblk2 : Outport
  wires:
  cfblk3/1 -> cfblk4/1
  cfblk6/1 -> cfblk3/1
  cfblk1/1 -> cfblk6/1
  cfblk4/1 -> cfblk2/1
  cfblk5/1 -> cfblk6/2
  cfblk7/1 -> cfblk5/1
  cfblk4/2 -> cfblk9/1
  cfblk9/1 -> cfblk6/3

== system sampleModel1000/cfblk125/cfblk8 ==
  cfblk1 : Inport
  cfblk9 : Inport  Port=2
  cfblk10 : Inport  Port=3
  cfblk3 : simulink/Math Operations/Slider Gain  gain=1  low=0  high=2
  cfblk4 : UnaryMinus
  cfblk5 : Constant  Value=[312453252.663151]  SampleTime=1
  cfblk6 : Constant  Value=[-148155631.933216]  SampleTime=1
  cfblk7 : Constant  Value=[-621626820.272362]  SampleTime=1
  cfblk8 : Constant  Value=[256908239.646860]  SampleTime=1
  cfblk2 : Outport
  cfblk11 : Outport  Port=2
  cfblk12 : Outport  Port=3
  cfblk13 : Outport  Port=4
  cfblk14 : Outport  Port=5
  cfblk15 : Outport  Port=6
  cfblk16 : Outport  Port=7
  wires:
  cfblk9/1 -> cfblk14/1
  cfblk3/1 -> cfblk16/1
  cfblk5/1 -> cfblk3/1
  cfblk8/1 -> cfblk12/1
  cfblk7/1 -> cfblk2/1
  cfblk1/1 -> cfblk15/1
  cfblk6/1 -> cfblk11/1
  cfblk4/1 -> cfblk13/1
  cfblk10/1 -> cfblk4/1

== system sampleModel1000/cfblk125/cfblk9 ==
  cfblk1 : Inport
  cfblk7 : Inport  Port=2
  cfblk10 : Delay  SampleTime=1
  cfblk3 : DiscreteZeroPole  Poles=[0 0.5]  Gain=1
  cfblk4 : Delay  DelayLengthSource=Input port  SampleTime=1
      settings: InputPortMap=u0,p1
  cfblk5 : DiscreteFilter  SampleTime=1
  cfblk6 : Product  Inputs=**
  cfblk2 : Outport
  cfblk8 : Outport  Port=2
  cfblk9 : Outport  Port=3
  wires:
  cfblk7/1 -> cfblk8/1
  cfblk3/1 -> cfblk6/1, cfblk6/2, cfblk10/1
  cfblk6/1 -> cfblk2/1
  cfblk5/1 -> cfblk3/1, cfblk9/1
  cfblk4/1 -> cfblk5/1
  cfblk1/1 -> cfblk4/1
  cfblk10/1 -> cfblk4/2

== system sampleModel1000/cfblk126/cfblk10 ==
  cfblk1 : Inport
  cfblk7 : Inport  Port=2
  cfblk3 : simulink/Discrete/Transfer Fcn Lead or Lag  PoleZ=0.95  ZeroZ=0.75  ICPrevOutput=0.0  ICPrevInput=0.0  DoSatur=off
      settings: SourceProductBaseCode=SL
  cfblk4 : Delay  ShowEnablePort=on  SampleTime=1
      settings: InputPortMap=u0,e6
  cfblk5 : Sum  Inputs=+-
  cfblk6 : Sum  Inputs=|++
  cfblk8 : Delay  SampleTime=1
  cfblk2 : Outport
  wires:
  cfblk6/1 -> cfblk2/1, cfblk4/2
  cfblk1/1 -> cfblk6/1
  cfblk3/1 -> cfblk6/2
  cfblk4/1 -> cfblk5/1
  cfblk7/1 -> cfblk5/2, cfblk3/1
  cfblk5/1 -> cfblk8/1
  cfblk8/1 -> cfblk4/1

== system sampleModel1000/cfblk127/cfblk10 ==
  cfblk1 : Inport
  cfblk3 : DiscreteIntegrator  ICPrevOutput=DiscIntNeverNeededParam  ICPrevScaledInput=DiscIntNeverNeededParam
  cfblk4 : simulink/Math Operations/MinMax Running Resettable  Function=min  vinit=0.0
  cfblk5 : Trigonometry
  cfblk6 : Constant  Value=[-746085580.429931]  SampleTime=1
  cfblk7 : Constant  Value=[-524679379.923421]  SampleTime=1
  cfblk2 : Outport
  wires:
  cfblk6/1 -> cfblk4/1
  cfblk5/1 -> cfblk3/1
  cfblk1/1 -> cfblk2/1
  cfblk4/1 -> cfblk5/1
  cfblk7/1 -> cfblk4/2

== system sampleModel1000/cfblk127/cfblk11 ==
  cfblk1 : Inport
  cfblk13 : Inport  Port=2
  cfblk14 : Inport  Port=3
  cfblk10 : Product  Inputs=*
  cfblk11 : Rounding
  cfblk12 : Constant  Value=[729150256.694984]  SampleTime=1
  cfblk16 : Delay  SampleTime=1
  cfblk3 : simulink/Discrete/Transfer Fcn Real Zero  ZeroZ=0.75  ICPrevInput=0.0  DoSatur=off
      settings: SourceProductBaseCode=SL
  cfblk4 : simulink/Discrete/Transfer Fcn Lead or Lag  PoleZ=0.95  ZeroZ=0.75  ICPrevOutput=0.0  ICPrevInput=0.0  DoSatur=off
      settings: SourceProductBaseCode=SL
  cfblk5 : UnitDelay  HasFrameUpgradeWarning=on
  cfblk6 : slpidlib/PID Controller  Controller=PID  Form=Parallel  TimeDomain=Discrete-time  UseExternalTs=off  SampleTime=1  IntegratorMethod=Forward Euler  FilterMethod=Forward Euler  ControllerParametersSource=internal  P=1  I=1  UseKiTs=off  D=0  N=100  UseFilter=on  TunerSelectOption=Transfer Function Based (PID Tuner App)  InitialConditionSource=internal  InitialConditionForIntegrator=0  InitialConditionForFilter=0  DifferentiatorICPrevScaledInput=0  ExternalReset=none  TrackingMode=off  Kt=1  LimitOutput=off  SatLimitsSource=internal  UpperSaturationLimit=inf  LowerSaturationLimit=-inf  LinearizeAsGain=off  AntiWindupMode=none  Kb=1  POutMin=[]  POutMax=[]  IOutMin=[]  IOutMax=[]  DOutMin=[]  DOutMax=[]  NOutMin=[]  NOutMax=[]  SumOutMin=[]  SumOutMax=[]  SaturationOutMin=[]  SaturationOutMax=[]  PParamMin=[]  PParamMax=[]  IParamMin=[]  IParamMax=[]  DParamMin=[]  DParamMax=[]  NParamMin=[]  NParamMax=[]  KbParamMin=[]  KbParamMax=[]  KtParamMin=[]  KtParamMax=[]  KbOutMin=[]  KbOutMax=[]  KtOutMin=[]  KtOutMax=[]  IntegratorOutMin=[]  IntegratorOutMax=[]  FilterOutMin=[]  FilterOutMax=[]  SumI1OutMin=[]  SumI1OutMax=[]  SumI2OutMin=[]  SumI2OutMax=[]  SumI3OutMin=[]  SumI3OutMax=[]  SumI4OutMin=[]  SumI4OutMax=[]  SumDOutMin=[]  SumDOutMax=[]  DifferentiatorOutMin=[]  DifferentiatorOutMax=[]  FilterDiffOutCoefMin=[]  FilterDiffOutCoefMax=[]  ReciprocalOutMin=[]  ReciprocalOutMax=[]  SumDenOutMin=[]  SumDenOutMax=[]  SumNumOutMin=[]  SumNumOutMax=[]  DivideOutMin=[]  DivideOutMax=[]  UdiffTsProdOutMin=[]  UdiffTsProdOutMax=[]  NTsProdOutMin=[]  NTsProdOutMax=[]  UintegralTsProdOutMin=[]  UintegralTsProdOutMax=[]  UngainTsProdOutMin=[]  UngainTsProdOutMax=[]  IntegratorContinuousStateAttributes=''  IntegratorStateMustResolveToSignalObject=off  IntegratorRTWStateStorageClass=Auto  FilterContinuousStateAttributes=''  FilterStateMustResolveToSignalObject=off  FilterRTWStateStorageClass=Auto  ParallelPVariant=InternalParameters  IdealPVariant=Disabled  IVariant=InternalParameters  DVariant=InternalParameters  IntegratorVariant=Discrete  SatVariant=Disabled  AWVariant=Passthrough  PCopyVariant=Disabled  TRVariant=Disabled  FdbkBlocksVariant=Forward  IdealPFdbkVariant=Disabled  SatFdbkVariant=Disabled  DerivativeFilterVariant=ForwardEulerFilter  NVariant=InternalParameters  NCopyVariant=Disabled  FilterICVariant=InternalICsFilter  IntegratorICVariant=InternalICs  ExternalResetVariant=Disabled  TRSumVariant=Passthrough  SumFdbkVariant=Disabled  SumVariant=Sum_PID  TsampFilterVariant=InternalTs  TsampNgainVariant=Passthrough  TsampIntegralVariant=Passthrough  ExternalSaturationOutDataTypeStr=Inherit: Same as second input  aMode=0
  cfblk7 : Product  Inputs=**
  cfblk8 : Assignment  DiagnosticForDimensions=Warning  IndexOptions=Index vector (dialog)  Indices=1  OutputSizes=1
  cfblk9 : simulink/Math Operations/MinMax Running Resettable  Function=min  vinit=0.0
  cfblk2 : Outport
  cfblk15 : Outport  Port=2
  wires:
  cfblk6/1 -> cfblk3/1
  cfblk8/1 -> cfblk2/1
  cfblk5/1 -> cfblk4/1
  cfblk1/1 -> cfblk6/1
  cfblk7/1 -> cfblk11/1
  cfblk13/1 -> cfblk7/1
  cfblk14/1 -> cfblk7/2, cfblk15/1
  cfblk4/1 -> cfblk9/1
  cfblk12/1 -> cfblk5/1
  cfblk11/1 -> cfblk8/1
  cfblk3/1 -> cfblk8/2
  cfblk9/1 -> cfblk10/1
  cfblk10/1 -> cfblk16/1
  cfblk16/1 -> cfblk9/2

== system sampleModel1000/cfblk127/cfblk12 ==
  cfblk1 : Inport
  cfblk12 : Inport  Port=2
  cfblk13 : Inport  Port=3
  cfblk10 : Constant  Value=[615128914.038853]  SampleTime=1
  cfblk11 : Constant  Value=[859922555.780517]  SampleTime=1
  cfblk15 : Delay  SampleTime=1
  cfblk3 : Delay  ShowEnablePort=on  SampleTime=1
      settings: InputPortMap=u0,e6
  cfblk4 : ComplexToMagnitudeAngle
  cfblk5 : Gain  Gain=[668982421.802994]
  cfblk6 : Sqrt  Operator=rSqrt  AlgorithmType=Newton-Raphson
  cfblk7 : simulink/Math Operations/MinMax Running Resettable  Function=min  vinit=0.0
  cfblk8 : Math  Operator=log
  cfblk9 : Product
  cfblk2 : Outport
  cfblk14 : Outport  Port=2
  wires:
  cfblk10/1 -> cfblk2/1
  cfblk1/1 -> cfblk5/1
  cfblk7/1 -> cfblk8/1
  cfblk8/1 -> cfblk6/1
  cfblk12/1 -> cfblk3/1
  cfblk5/1 -> cfblk3/2
  cfblk11/1 -> cfblk9/1
  cfblk3/1 -> cfblk14/1
  cfblk4/1 -> cfblk9/2
  cfblk4/2 -> cfblk7/1
  cfblk13/1 -> cfblk7/2
  cfblk6/1 -> cfblk15/1
  cfblk15/1 -> cfblk4/1

== system sampleModel1000/cfblk127/cfblk18 ==
  cfblk1 : Inport
  cfblk15 : Inport  Port=2
  Action Port : ActionPort  ActionPortLabel=if(u1 >= 0)
  cfblk10 : Product  Inputs=*
  cfblk11 : Product
  cfblk12 : Sqrt
  cfblk13 : Constant  Value=[793281884.610753]  SampleTime=1
  cfblk14 : Constant  Value=[227386444.303892]  SampleTime=1
  cfblk17 : Delay
  cfblk3 : simulink/Discrete/Transfer Fcn Real Zero  ZeroZ=0.75  ICPrevInput=0.0  DoSatur=off
      settings: SourceProductBaseCode=SL
  cfblk4 : slpidlib/PID Controller (2DOF)  Controller=PID  Form=Parallel  TimeDomain=Discrete-time  UseExternalTs=off  SampleTime=-1  IntegratorMethod=Forward Euler  FilterMethod=Forward Euler  ControllerParametersSource=internal  P=1  I=1  UseKiTs=off  D=0  N=100  UseFilter=on  b=1  c=1  TunerSelectOption=Transfer Function Based (PID Tuner App)  InitialConditionSource=internal  InitialConditionForIntegrator=0  InitialConditionForFilter=0  DifferentiatorICPrevScaledInput=0  ExternalReset=none  TrackingMode=off  Kt=1  LimitOutput=off  SatLimitsSource=internal  UpperSaturationLimit=inf  LowerSaturationLimit=-inf  LinearizeAsGain=off  AntiWindupMode=none  Kb=1  POutMin=[]  POutMax=[]  IOutMin=[]  IOutMax=[]  DOutMin=[]  DOutMax=[]  NOutMin=[]  NOutMax=[]  bOutMin=[]  bOutMax=[]  cOutMin=[]  cOutMax=[]  SumOutMin=[]  SumOutMax=[]  SaturationOutMin=[]  SaturationOutMax=[]  PParamMin=[]  PParamMax=[]  IParamMin=[]  IParamMax=[]  DParamMin=[]  DParamMax=[]  NParamMin=[]  NParamMax=[]  bParamMin=[]  bParamMax=[]  cParamMin=[]  cParamMax=[]  KbParamMin=[]  KbParamMax=[]  KtParamMin=[]  KtParamMax=[]  KbOutMin=[]  KbOutMax=[]  KtOutMin=[]  KtOutMax=[]  IntegratorOutMin=[]  IntegratorOutMax=[]  FilterOutMin=[]  FilterOutMax=[]  SumI1OutMin=[]  SumI1OutMax=[]  SumI2OutMin=[]  SumI2OutMax=[]  SumI3OutMin=[]  SumI3OutMax=[]  SumI4OutMin=[]  SumI4OutMax=[]  SumDOutMin=[]  SumDOutMax=[]  Sum1OutMin=[]  Sum1OutMax=[]  Sum2OutMin=[]  Sum2OutMax=[]  Sum3OutMin=[]  Sum3OutMax=[]  DifferentiatorOutMin=[]  DifferentiatorOutMax=[]  FilterDiffOutCoefMin=[]  FilterDiffOutCoefMax=[]  ReciprocalOutMin=[]  ReciprocalOutMax=[]  SumDenOutMin=[]  SumDenOutMax=[]  SumNumOutMin=[]  SumNumOutMax=[]  DivideOutMin=[]  DivideOutMax=[]  UdiffTsProdOutMin=[]  UdiffTsProdOutMax=[]  NTsProdOutMin=[]  NTsProdOutMax=[]  UintegralTsProdOutMin=[]  UintegralTsProdOutMax=[]  UngainTsProdOutMin=[]  UngainTsProdOutMax=[]  IntegratorContinuousStateAttributes=''  IntegratorStateMustResolveToSignalObject=off  IntegratorRTWStateStorageClass=Auto  FilterContinuousStateAttributes=''  FilterStateMustResolveToSignalObject=off  FilterRTWStateStorageClass=Auto  ParallelPVariant=InternalParameters  IdealPVariant=Disabled  IVariant=InternalParameters  DVariant=InternalParameters  bVariant=InternalParameters  cVariant=InternalParameters  IntegratorVariant=Discrete  SatVariant=Disabled  AWVariant=Passthrough  PCopyVariant=Disabled  TRVariant=Disabled  FdbkBlocksVariant=Forward  IdealPFdbkVariant=Disabled  SatFdbkVariant=Disabled  DerivativeFilterVariant=ForwardEulerFilter  NVariant=InternalParameters  NCopyVariant=Disabled  FilterICVariant=InternalICsFilter  IntegratorICVariant=InternalICs  ExternalResetVariant=Disabled  TRSumVariant=Passthrough  SumFdbkVariant=Disabled  SumVariant=Sum_PID  TsampFilterVariant=InternalTs  TsampNgainVariant=Passthrough  TsampIntegralVariant=Passthrough  ExternalSaturationOutDataTypeStr=Inherit: Same as second input
      settings: SourceProductBaseCode=SL
  cfblk5 : DiscreteFilter
  cfblk6 : simulink/Discrete/Tapped Delay  vinit=0.0  samptime=-1  NumDelays=1  DelayOrder=Oldest  includeCurrent=off
  cfblk7 : simulink/Discrete/Transfer Fcn Lead or Lag  PoleZ=0.95  ZeroZ=0.75  ICPrevOutput=0.0  ICPrevInput=0.0  DoSatur=off
      settings: SourceProductBaseCode=SL
  cfblk8 : DiscreteFir
  cfblk9 : simulink/Math Operations/MinMax Running Resettable  Function=min  vinit=0.0
  cfblk2 : Outport
  cfblk16 : Outport  Port=2
  wires:
  cfblk4/1 -> cfblk3/1
  cfblk12/1 -> cfblk9/1
  cfblk11/1 -> cfblk12/1
  cfblk13/1 -> cfblk2/1, cfblk11/2
  cfblk6/1 -> cfblk4/1
  cfblk3/1 -> cfblk7/1
  cfblk14/1 -> cfblk4/2
  cfblk8/1 -> cfblk16/1
  cfblk9/1 -> cfblk6/1
  cfblk7/1 -> cfblk10/1
  cfblk15/1 -> cfblk5/1
  cfblk1/1 -> cfblk11/1
  cfblk5/1 -> cfblk8/1
  cfblk10/1 -> cfblk17/1
  cfblk17/1 -> cfblk9/2

== system sampleModel1000/cfblk127/cfblk19 ==
  cfblk1 : Inport
  cfblk14 : Inport  Port=2
  Action Port : ActionPort  ActionPortLabel=else
  cfblk10 : MinMax  Inputs=3
  cfblk11 : Assignment  DiagnosticForDimensions=Warning  IndexOptions=Index vector (dialog)  Indices=1  OutputSizes=1
  cfblk12 : Constant  Value=[750015721.770692]  SampleTime=1
  cfblk13 : Constant  Value=[857367764.681765]  SampleTime=1
  cfblk16 : Delay
  cfblk17 : Delay
  cfblk3 : simulink/Discrete/Transfer Fcn Lead or Lag  PoleZ=0.95  ZeroZ=0.75  ICPrevOutput=0.0  ICPrevInput=0.0  DoSatur=off
      settings: SourceProductBaseCode=SL
  cfblk4 : Delay  ShowEnablePort=on
      settings: InputPortMap=u0,e6
  cfblk5 : slpidlib/PID Controller (2DOF)  Controller=PID  Form=Parallel  TimeDomain=Discrete-time  UseExternalTs=off  SampleTime=-1  IntegratorMethod=Forward Euler  FilterMethod=Forward Euler  ControllerParametersSource=internal  P=1  I=1  UseKiTs=off  D=0  N=100  UseFilter=on  b=1  c=1  TunerSelectOption=Transfer Function Based (PID Tuner App)  InitialConditionSource=internal  InitialConditionForIntegrator=0  InitialConditionForFilter=0  DifferentiatorICPrevScaledInput=0  ExternalReset=none  TrackingMode=off  Kt=1  LimitOutput=off  SatLimitsSource=internal  UpperSaturationLimit=inf  LowerSaturationLimit=-inf  LinearizeAsGain=off  AntiWindupMode=none  Kb=1  POutMin=[]  POutMax=[]  IOutMin=[]  IOutMax=[]  DOutMin=[]  DOutMax=[]  NOutMin=[]  NOutMax=[]  bOutMin=[]  bOutMax=[]  cOutMin=[]  cOutMax=[]  SumOutMin=[]  SumOutMax=[]  SaturationOutMin=[]  SaturationOutMax=[]  PParamMin=[]  PParamMax=[]  IParamMin=[]  IParamMax=[]  DParamMin=[]  DParamMax=[]  NParamMin=[]  NParamMax=[]  bParamMin=[]  bParamMax=[]  cParamMin=[]  cParamMax=[]  KbParamMin=[]  KbParamMax=[]  KtParamMin=[]  KtParamMax=[]  KbOutMin=[]  KbOutMax=[]  KtOutMin=[]  KtOutMax=[]  IntegratorOutMin=[]  IntegratorOutMax=[]  FilterOutMin=[]  FilterOutMax=[]  SumI1OutMin=[]  SumI1OutMax=[]  SumI2OutMin=[]  SumI2OutMax=[]  SumI3OutMin=[]  SumI3OutMax=[]  SumI4OutMin=[]  SumI4OutMax=[]  SumDOutMin=[]  SumDOutMax=[]  Sum1OutMin=[]  Sum1OutMax=[]  Sum2OutMin=[]  Sum2OutMax=[]  Sum3OutMin=[]  Sum3OutMax=[]  DifferentiatorOutMin=[]  DifferentiatorOutMax=[]  FilterDiffOutCoefMin=[]  FilterDiffOutCoefMax=[]  ReciprocalOutMin=[]  ReciprocalOutMax=[]  SumDenOutMin=[]  SumDenOutMax=[]  SumNumOutMin=[]  SumNumOutMax=[]  DivideOutMin=[]  DivideOutMax=[]  UdiffTsProdOutMin=[]  UdiffTsProdOutMax=[]  NTsProdOutMin=[]  NTsProdOutMax=[]  UintegralTsProdOutMin=[]  UintegralTsProdOutMax=[]  UngainTsProdOutMin=[]  UngainTsProdOutMax=[]  IntegratorContinuousStateAttributes=''  IntegratorStateMustResolveToSignalObject=off  IntegratorRTWStateStorageClass=Auto  FilterContinuousStateAttributes=''  FilterStateMustResolveToSignalObject=off  FilterRTWStateStorageClass=Auto  ParallelPVariant=InternalParameters  IdealPVariant=Disabled  IVariant=InternalParameters  DVariant=InternalParameters  bVariant=InternalParameters  cVariant=InternalParameters  IntegratorVariant=Discrete  SatVariant=Disabled  AWVariant=Passthrough  PCopyVariant=Disabled  TRVariant=Disabled  FdbkBlocksVariant=Forward  IdealPFdbkVariant=Disabled  SatFdbkVariant=Disabled  DerivativeFilterVariant=ForwardEulerFilter  NVariant=InternalParameters  NCopyVariant=Disabled  FilterICVariant=InternalICsFilter  IntegratorICVariant=InternalICs  ExternalResetVariant=Disabled  TRSumVariant=Passthrough  SumFdbkVariant=Disabled  SumVariant=Sum_PID  TsampFilterVariant=InternalTs  TsampNgainVariant=Passthrough  TsampIntegralVariant=Passthrough  ExternalSaturationOutDataTypeStr=Inherit: Same as second input
      settings: SourceProductBaseCode=SL
  cfblk6 : simulink/Discrete/Transfer Fcn First Order  PoleZ=0.95  ICPrevOutput=0.0  DoSatur=off
  cfblk7 : ComplexToMagnitudeAngle
  cfblk8 : Trigonometry
  cfblk9 : Math  Operator=pow
  cfblk2 : Outport
  cfblk15 : Outport  Port=2
  wires:
  cfblk6/1 -> cfblk16/1, cfblk17/1
  cfblk7/1 -> cfblk9/1
  cfblk5/1 -> cfblk4/1
  cfblk10/1 -> cfblk8/1
  cfblk4/1 -> cfblk7/1
  cfblk1/1 -> cfblk5/2, cfblk4/2
  cfblk7/2 -> cfblk10/1, cfblk9/2
  cfblk14/1 -> cfblk11/1
  cfblk12/1 -> cfblk2/1
  cfblk8/1 -> cfblk6/1
  cfblk11/1 -> cfblk15/1
  cfblk3/1 -> cfblk10/2
  cfblk13/1 -> cfblk3/1
  cfblk9/1 -> cfblk11/2
  cfblk16/1 -> cfblk5/1
  cfblk17/1 -> cfblk10/3

== system sampleModel1000/cfblk127/cfblk9 ==
  cfblk1 : Inport
  cfblk8 : Inport  Port=2
  cfblk9 : Inport  Port=3
  cfblk10 : Inport  Port=4
  cfblk3 : Delay  DelayLengthSource=Input port  SampleTime=1
      settings: InputPortMap=u0,p1
  cfblk4 : simulink/Discrete/Transfer Fcn First Order  PoleZ=0.95  ICPrevOutput=0.0  DoSatur=off
  cfblk5 : MinMax
  cfblk6 : Sum  Inputs=|++
  cfblk7 : Sqrt  Operator=rSqrt  AlgorithmType=Newton-Raphson
  cfblk2 : Outport
  wires:
  cfblk8/1 -> cfblk3/1
  cfblk9/1 -> cfblk6/1
  cfblk10/1 -> cfblk4/1
  cfblk6/1 -> cfblk7/1
  cfblk7/1 -> cfblk2/1
  cfblk1/1 -> cfblk6/2
  cfblk4/1 -> cfblk3/2
  cfblk3/1 -> cfblk5/1

== system sampleModel1000/cfblk128/cfblk10 ==
  cfblk1 : Inport
  cfblk11 : Inport  Port=2
  cfblk12 : Inport  Port=3
  cfblk13 : Inport  Port=4
  cfblk10 : Constant  Value=[-502659713.459819]  SampleTime=1
  cfblk3 : DiscreteIntegrator  ICPrevOutput=DiscIntNeverNeededParam  ICPrevScaledInput=DiscIntNeverNeededParam
  cfblk4 : simulink/Discrete/Transfer Fcn Real Zero  ZeroZ=0.75  ICPrevInput=0.0  DoSatur=off
      settings: SourceProductBaseCode=SL
  cfblk5 : UnitDelay  HasFrameUpgradeWarning=on
  cfblk6 : DiscreteZeroPole  Poles=[0 0.5]  Gain=1
  cfblk7 : Abs  SaturateOnIntegerOverflow=off
  cfblk8 : Sum  Inputs=|++
  cfblk9 : Sqrt
  cfblk2 : Outport
  cfblk14 : Outport  Port=2
  wires:
  cfblk13/1 -> cfblk3/1
  cfblk6/1 -> cfblk7/1
  cfblk8/1 -> cfblk4/1
  cfblk11/1 -> cfblk9/1
  cfblk5/1 -> cfblk14/1
  cfblk7/1 -> cfblk8/1
  cfblk9/1 -> cfblk6/1
  cfblk12/1 -> cfblk5/1
  cfblk4/1 -> cfblk2/1
  cfblk3/1 -> cfblk8/2

== system sampleModel1000/cfblk128/cfblk11 ==
  cfblk1 : Inport
  cfblk11 : Delay  SampleTime=1
  cfblk12 : Delay  SampleTime=1
  cfblk3 : simulink/Discrete/Transfer Fcn First Order  PoleZ=0.95  ICPrevOutput=0.0  DoSatur=off
  cfblk4 : Delay  DelayLengthSource=Input port  SampleTime=1
      settings: InputPortMap=u0,p1
  cfblk5 : simulink/Discrete/Difference  ICPrevInput=0.0  OutMin=[]  OutMax=[]  OutDataTypeStr=Inherit: Inherit via back propagation  OutDataType=fixdt(1, 16)  OutScaling=2^-10  DoSatur=off
  cfblk6 : simulink/Discrete/Transfer Fcn Real Zero  ZeroZ=0.75  ICPrevInput=0.0  DoSatur=off
      settings: SourceProductBaseCode=SL
  cfblk7 : Reshape
  cfblk8 : Sum  Inputs=|++
  cfblk9 : Constant  Value=[14854266.189556]  SampleTime=1
  cfblk2 : Outport
  cfblk10 : Outport  Port=2
  wires:
  cfblk4/1 -> cfblk7/1, cfblk10/1
  cfblk9/1 -> cfblk2/1
  cfblk8/1 -> cfblk4/1
  cfblk1/1 -> cfblk6/1
  cfblk6/1 -> cfblk3/1
  cfblk7/1 -> cfblk5/1, cfblk11/1
  cfblk3/1 -> cfblk8/2
  cfblk11/1 -> cfblk4/2
  cfblk5/1 -> cfblk12/1
  cfblk12/1 -> cfblk8/1
